simulink library "Battery_Cell_Det"  (R2014a)
settings: Solver=ode45  StartTime=0.0  StopTime=10.0  RelTol=1e-3
undefined symbols (not defined in the file): HEV_Param, Kt_Temps
libraries: fl_lib x18, LeadAcidBattery_lib x12, nesl_utility x3
Description:
  | Copyright 2014 The MathWorks, Inc.
settings Model: Creator=smiller  LastModifiedBy=psanghvi

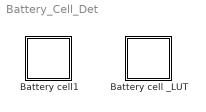
== system Battery_Cell_Det ==
  Battery cell _LUT : Subsystem
      mask Display:
      | image(imread('battery.jpg'))
      | color('red')
      | port_label('LConn',1,'H')
      | port_label('LConn',2,'+')
      | port_label('RConn',1,'-')
  Battery cell1 : Subsystem
      mask Display:
      | image(imread('battery.jpg'))
      | color('red')
      | port_label('LConn',1,'H')
      | port_label('LConn',2,'+')
      | port_label('RConn',1,'-')

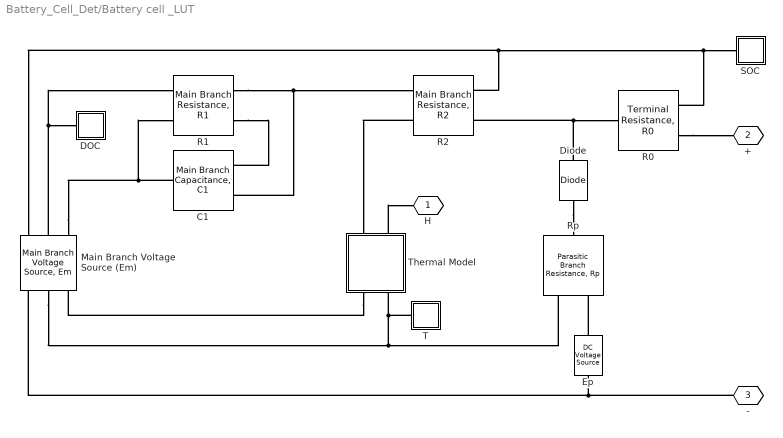
== system Battery_Cell_Det/Battery cell _LUT ==
  " DOC " : Subsystem
  " SOC " : Subsystem
  C1 : LeadAcidBattery_lib/Main Branch Capacitance, C1  Tau1=HEV_Param.Battery_Cell.Tau1 s  Cmin=1e-5 F
  Diode : fl_lib/Electrical/Electrical Elements/Diode  Vf=0.6 V  Ron=0.3 Ohm  Goff=1e-08 1/Ohm  i_specify=off  i_priority=High  i=0 A  v_specify=off  v_priority=High  v=0 V
  Ep : fl_lib/Electrical/Electrical Sources/DC Voltage Source  v0=HEV_Param.Battery_Cell.Ep V
  Main Branch Voltage Source (Em) : LeadAcidBattery_lib/Main Branch Voltage Source, Em  Em0=HEV_Param.Battery_Cell.Emo V  Ke=HEV_Param.Battery_Cell.Ke V/K  Kc=HEV_Param.Battery_Cell.Kc  C0=HEV_Param.Battery_Cell.Costar s*A  Istar=HEV_Param.Battery_Cell.Istar A  delta=HEV_Param.Battery_Cell.delta  Tau1=HEV_Param.Battery_Cell.Tau1 s  Qinit=HEV_Param.Battery_Cell.Qe_init s*A
  R0 : LeadAcidBattery_lib/Terminal Resistance, R0  R00=HEV_Param.Battery_Cell.Roo Ohm  A0=HEV_Param.Battery_Cell.Ao
  R1 : LeadAcidBattery_lib/Main Branch Resistance, R1  R10=HEV_Param.Battery_Cell.R10 Ohm  DOC_min=1e-006
  R2 : LeadAcidBattery_lib/Main Branch Resistance, R2  R20=HEV_Param.Battery_Cell.R20 Ohm  A21=HEV_Param.Battery_Cell.A21  A22=HEV_Param.Battery_Cell.A22  Istar=HEV_Param.Battery_Cell.Istar A
  Rp : LeadAcidBattery_lib/Parasitic Branch Resistance, Rp  Gp0=HEV_Param.Battery_Cell.Gpo 1/Ohm  Vp0=HEV_Param.Battery_Cell.Vpo V  Ap=HEV_Param.Battery_Cell.Ap  Tf=HEV_Param.Battery_Cell.theta_f C
  T : Subsystem
  Thermal Model : Subsystem
  H : PMIOPort  Tag=PMCPort  Port=1  Side=Left
  + : PMIOPort  Tag=PMCPort  Port=2  Side=Left
  - : PMIOPort  Tag=PMCPort  Port=3  Side=Right
  connections:
  Diode/LConn1 -- R0/RConn1 -- R2/LConn2
  R2/RConn2 -- Thermal Model/LConn1
  -/RConn1 -- Ep/RConn1 -- Main Branch Voltage Source (Em)/RConn1
  Thermal Model/RConn1 -- Main Branch Voltage Source (Em)/RConn3
  Diode/RConn1 -- Rp/LConn1
  Ep/LConn1 -- Rp/RConn2
  Thermal Model/LConn2 -- H/RConn1
  R2/LConn1 -- Main Branch Voltage Source (Em)/LConn1 -- R0/LConn1 -- " SOC "/LConn1
  R1/LConn2 -- C1/LConn1
  R1/LConn1 -- C1/LConn2 -- R2/RConn1
  Main Branch Voltage Source (Em)/LConn3 -- C1/RConn1 -- R1/RConn2
  Main Branch Voltage Source (Em)/LConn2 -- R1/RConn1 -- " DOC "/LConn1
  R0/LConn2 -- +/RConn1
  Main Branch Voltage Source (Em)/RConn2 -- Rp/RConn1 -- T/LConn1 -- Thermal Model/RConn2

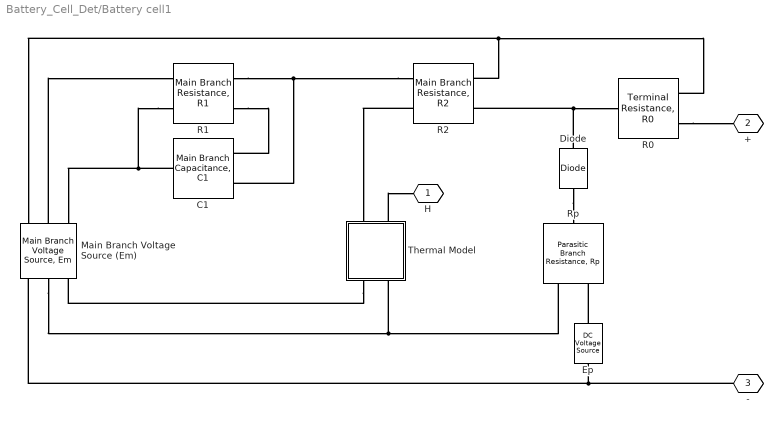
== system Battery_Cell_Det/Battery cell1 ==
  C1 : LeadAcidBattery_lib/Main Branch Capacitance, C1  Tau1=HEV_Param.Battery_Cell.Tau1 s  Cmin=1e-5 F
  Diode : fl_lib/Electrical/Electrical Elements/Diode  Vf=0.6 V  Ron=0.3 Ohm  Goff=1e-08 1/Ohm  i_specify=off  i_priority=High  i=0 A  v_specify=off  v_priority=High  v=0 V
  Ep : fl_lib/Electrical/Electrical Sources/DC Voltage Source  v0=HEV_Param.Battery_Cell.Ep V
  Main Branch Voltage Source (Em) : LeadAcidBattery_lib/Main Branch Voltage Source, Em  Em0=HEV_Param.Battery_Cell.Emo V  Ke=HEV_Param.Battery_Cell.Ke V/K  Kc=HEV_Param.Battery_Cell.Kc  C0=HEV_Param.Battery_Cell.Costar s*A  Istar=HEV_Param.Battery_Cell.Istar A  delta=HEV_Param.Battery_Cell.delta  Tau1=HEV_Param.Battery_Cell.Tau1 s  Qinit=HEV_Param.Battery_Cell.Qe_init s*A
  R0 : LeadAcidBattery_lib/Terminal Resistance, R0  R00=HEV_Param.Battery_Cell.Roo Ohm  A0=HEV_Param.Battery_Cell.Ao
  R1 : LeadAcidBattery_lib/Main Branch Resistance, R1  R10=HEV_Param.Battery_Cell.R10 Ohm  DOC_min=1e-006
  R2 : LeadAcidBattery_lib/Main Branch Resistance, R2  R20=HEV_Param.Battery_Cell.R20 Ohm  A21=HEV_Param.Battery_Cell.A21  A22=HEV_Param.Battery_Cell.A22  Istar=HEV_Param.Battery_Cell.Istar A
  Rp : LeadAcidBattery_lib/Parasitic Branch Resistance, Rp  Gp0=HEV_Param.Battery_Cell.Gpo 1/Ohm  Vp0=HEV_Param.Battery_Cell.Vpo V  Ap=HEV_Param.Battery_Cell.Ap  Tf=HEV_Param.Battery_Cell.theta_f C
  Thermal Model : Subsystem
  H : PMIOPort  Tag=PMCPort  Port=1  Side=Left
  + : PMIOPort  Tag=PMCPort  Port=2  Side=Left
  - : PMIOPort  Tag=PMCPort  Port=3  Side=Right
  connections:
  Thermal Model/RConn2 -- Rp/RConn1 -- Main Branch Voltage Source (Em)/RConn2
  R0/LConn2 -- +/RConn1
  Main Branch Voltage Source (Em)/LConn2 -- R1/RConn1
  R1/RConn2 -- C1/RConn1 -- Main Branch Voltage Source (Em)/LConn3
  R2/RConn1 -- C1/LConn2 -- R1/LConn1
  R1/LConn2 -- C1/LConn1
  R0/LConn1 -- Main Branch Voltage Source (Em)/LConn1 -- R2/LConn1
  Thermal Model/LConn2 -- H/RConn1
  Ep/LConn1 -- Rp/RConn2
  Diode/RConn1 -- Rp/LConn1
  Thermal Model/RConn1 -- Main Branch Voltage Source (Em)/RConn3
  Main Branch Voltage Source (Em)/RConn1 -- Ep/RConn1 -- -/RConn1
  R2/RConn2 -- Thermal Model/LConn1
  R2/LConn2 -- R0/RConn1 -- Diode/LConn1

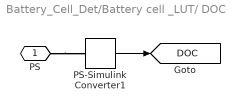
== system Battery_Cell_Det/Battery cell _LUT/ DOC  ==
  PS-Simulink Converter1 : nesl_utility/PS-Simulink Converter  PhysicalDomain=network_engine_domain  SubClassName=ps_output  LeftPortType=input  RightPortType=output  PseudoPeriodic=off  Frequencies=[]  Unit=1  AffineConversion=off
  PS : PMIOPort  Port=1  Side=Left
  tag scope: DOC=global
  wires:
  PS-Simulink Converter1/1 -> [DOC]
  connections:
  PS/RConn1 -- PS-Simulink Converter1/LConn1

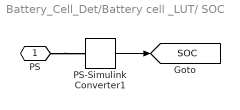
== system Battery_Cell_Det/Battery cell _LUT/ SOC  ==
  PS-Simulink Converter1 : nesl_utility/PS-Simulink Converter  PhysicalDomain=network_engine_domain  SubClassName=ps_output  LeftPortType=input  RightPortType=output  PseudoPeriodic=off  Frequencies=[]  Unit=1  AffineConversion=off
  PS : PMIOPort  Port=1  Side=Left
  tag scope: SOC=global
  wires:
  PS-Simulink Converter1/1 -> [SOC]
  connections:
  PS/RConn1 -- PS-Simulink Converter1/LConn1

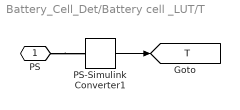
== system Battery_Cell_Det/Battery cell _LUT/T ==
  PS-Simulink Converter1 : nesl_utility/PS-Simulink Converter  PhysicalDomain=network_engine_domain  SubClassName=ps_output  LeftPortType=input  RightPortType=output  PseudoPeriodic=off  Frequencies=[]  Unit=C  AffineConversion=on
  PS : PMIOPort  Port=1  Side=Left
  tag scope: T=global
  wires:
  PS-Simulink Converter1/1 -> [T]
  connections:
  PS/RConn1 -- PS-Simulink Converter1/LConn1

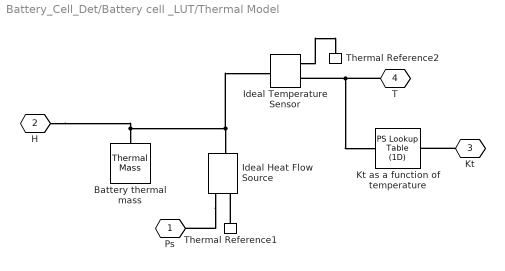
== system Battery_Cell_Det/Battery cell _LUT/Thermal Model ==
  Battery thermal mass : fl_lib/Thermal/Thermal Elements/Thermal Mass  mass=1 kg  sp_heat=HEV_Param.Battery_Cell.Ctheta J/kg/K  Q_specify=off  Q_priority=High  Q=0 J/s  T_specify=on  T_priority=High  T=HEV_Param.Battery_Cell.theta_init+273 K
  Ideal Temperature Sensor : fl_lib/Thermal/Thermal Sensors/Ideal Temperature Sensor
  Ideal Heat Flow Source : fl_lib/Thermal/Thermal Sources/Ideal Heat Flow Source
  Kt as a function of temperature : fl_lib/Physical Signals/Lookup Tables/PS Lookup Table (1D)  x_t=[HEV_Param.Battery_Cell.theta_f,HEV_Param.Battery_Cell. Kt_Temps]+273  y_t=[0 HEV_Param.Battery_Cell.Kt]  interp_method=1  extrap_method=1
  Thermal Reference1 : fl_lib/Thermal/Thermal Elements/Thermal Reference
  Thermal Reference2 : fl_lib/Thermal/Thermal Elements/Thermal Reference
  Ps : PMIOPort  Tag=PMCPort  Port=1  Side=Left
  H : PMIOPort  Tag=PMCPort  Port=2  Side=Left
  Kt : PMIOPort  Tag=PMCPort  Port=3  Side=Right
  T : PMIOPort  Tag=PMCPort  Port=4  Side=Right
  connections:
  Ideal Heat Flow Source/RConn1 -- Ps/RConn1
  Kt/RConn1 -- Kt as a function of temperature/RConn1
  Battery thermal mass/LConn1 -- Ideal Heat Flow Source/LConn1 -- Ideal Temperature Sensor/LConn1 -- H/RConn1
  Thermal Reference1/LConn1 -- Ideal Heat Flow Source/RConn2
  T/RConn1 -- Kt as a function of temperature/LConn1 -- Ideal Temperature Sensor/RConn2
  Ideal Temperature Sensor/RConn1 -- Thermal Reference2/LConn1

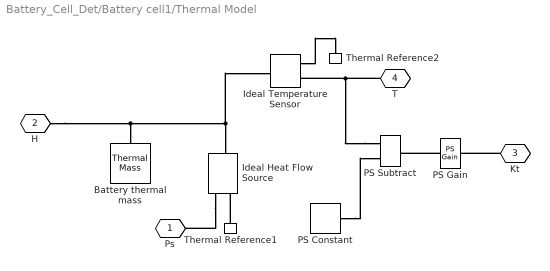
== system Battery_Cell_Det/Battery cell1/Thermal Model ==
  Battery thermal mass : fl_lib/Thermal/Thermal Elements/Thermal Mass  mass=1 kg  sp_heat=HEV_Param.Battery_Cell.Ctheta J/kg/K  Q_specify=off  Q_priority=High  Q=0 J/s  T_specify=on  T_priority=High  T=HEV_Param.Battery_Cell.theta_init+273 K
  Ideal Temperature Sensor : fl_lib/Thermal/Thermal Sensors/Ideal Temperature Sensor
  Ideal Heat Flow Source : fl_lib/Thermal/Thermal Sources/Ideal Heat Flow Source
  PS Constant : fl_lib/Physical Signals/Sources/PS Constant  constant=2.89
  PS Gain : fl_lib/Physical Signals/Functions/PS Gain  gain=0.0123
  PS Subtract : fl_lib/Physical Signals/Functions/PS Subtract
  Thermal Reference1 : fl_lib/Thermal/Thermal Elements/Thermal Reference
  Thermal Reference2 : fl_lib/Thermal/Thermal Elements/Thermal Reference
  Ps : PMIOPort  Tag=PMCPort  Port=1  Side=Left
  H : PMIOPort  Tag=PMCPort  Port=2  Side=Left
  Kt : PMIOPort  Tag=PMCPort  Port=3  Side=Right
  T : PMIOPort  Tag=PMCPort  Port=4  Side=Right
  connections:
  Ideal Temperature Sensor/RConn1 -- Thermal Reference2/LConn1
  PS Subtract/LConn1 -- Ideal Temperature Sensor/RConn2 -- T/RConn1
  Thermal Reference1/LConn1 -- Ideal Heat Flow Source/RConn2
  H/RConn1 -- Ideal Temperature Sensor/LConn1 -- Ideal Heat Flow Source/LConn1 -- Battery thermal mass/LConn1
  Kt/RConn1 -- PS Gain/RConn1
  Ideal Heat Flow Source/RConn1 -- Ps/RConn1
  PS Constant/RConn1 -- PS Subtract/LConn2
  PS Gain/LConn1 -- PS Subtract/RConn1
